simulink model "gm_HDL_pfc_gold_fi_vnl"  (R2024b)
settings: Solver=FixedStepDiscrete  StartTime=0.0  StopTime=.4  RelTol=1e-3
InitFcn:
  | fidelity_pfc_vals;
  | load('C:\Users\Angel\Desktop\hil\pfc3ph\matlab\sim\sschdl\pfc_desktop\stateSpaceParameters.mat');
undefined symbols (not defined in the file or in its folder): a, b, c, DiscIntNeverNeededParam, Down, Gs, s, stateSpaceParameters_1, t_ss, tsw, Up
libraries: simulink x32, hdlmdlgenlib x24, hdlsllib x8, eePwmGenerator x3, dspsrcs4 x3, hdlssclib x2, simulink_need_slupdate x1
(part 3 of 4)

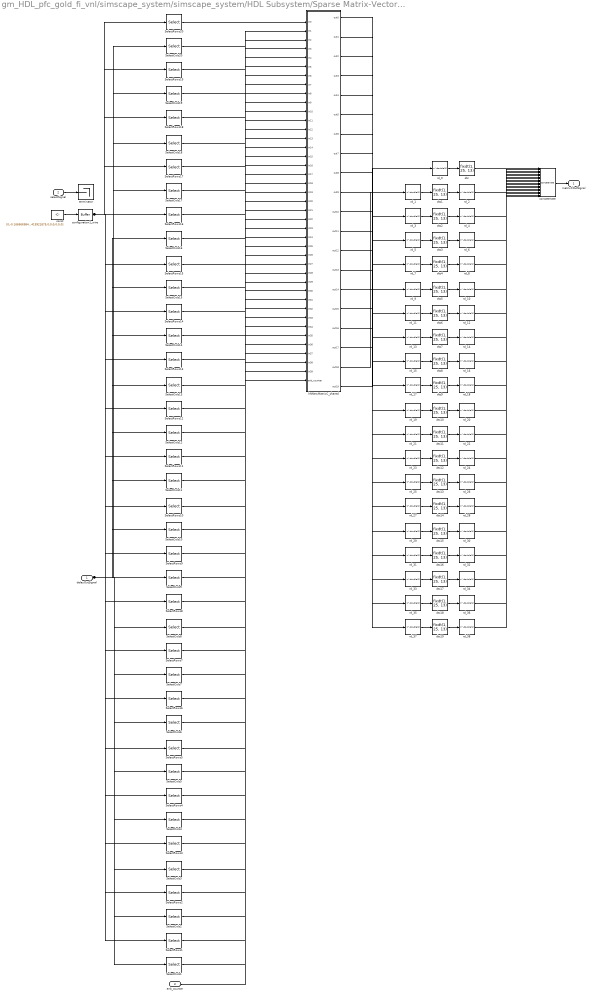
== system gm_HDL_pfc_gold_fi_vnl/simscape_system/simscape_system/HDL Subsystem/Sparse Matrix-Vector Product2 ==
  delayOutSignal : Inport  OutDataTypeStr=fixdt(1, 25, 13)  PortDimensions=[7]  SampleTime=7.65403750478377e-09
  selectSignal : Inport  Port=2  OutDataTypeStr=boolean  SampleTime=7.65403750478377e-09
  enb_counter : Inport  Port=3  OutDataTypeStr=fixdt(0, 7, 0)  SampleTime=7.65403750478377e-09
  SelectCols{1..20} (20 alike) : Selector  InputPortWidth=7  IndexOptions=Index vector (dialog)  Indices=double([1 2 3 4 5 6 7])  OutputSizes=double(1)
  SelectRows1 : Selector  InputPortWidth=140  IndexOptions=Index vector (dialog)  Indices=double([1 21 41 61 81 101 121])  OutputSizes=double(1)
  SelectRows10 : Selector  InputPortWidth=140  IndexOptions=Index vector (dialog)  Indices=double([10 30 50 70 90 110 130])  OutputSizes=double(1)
  SelectRows11 : Selector  InputPortWidth=140  IndexOptions=Index vector (dialog)  Indices=double([11 31 51 71 91 111 131])  OutputSizes=double(1)
  SelectRows12 : Selector  InputPortWidth=140  IndexOptions=Index vector (dialog)  Indices=double([12 32 52 72 92 112 132])  OutputSizes=double(1)
  SelectRows13 : Selector  InputPortWidth=140  IndexOptions=Index vector (dialog)  Indices=double([13 33 53 73 93 113 133])  OutputSizes=double(1)
  SelectRows14 : Selector  InputPortWidth=140  IndexOptions=Index vector (dialog)  Indices=double([14 34 54 74 94 114 134])  OutputSizes=double(1)
  SelectRows15 : Selector  InputPortWidth=140  IndexOptions=Index vector (dialog)  Indices=double([15 35 55 75 95 115 135])  OutputSizes=double(1)
  SelectRows16 : Selector  InputPortWidth=140  IndexOptions=Index vector (dialog)  Indices=double([16 36 56 76 96 116 136])  OutputSizes=double(1)
  SelectRows17 : Selector  InputPortWidth=140  IndexOptions=Index vector (dialog)  Indices=double([17 37 57 77 97 117 137])  OutputSizes=double(1)
  SelectRows18 : Selector  InputPortWidth=140  IndexOptions=Index vector (dialog)  Indices=double([18 38 58 78 98 118 138])  OutputSizes=double(1)
  SelectRows19 : Selector  InputPortWidth=140  IndexOptions=Index vector (dialog)  Indices=double([19 39 59 79 99 119 139])  OutputSizes=double(1)
  SelectRows2 : Selector  InputPortWidth=140  IndexOptions=Index vector (dialog)  Indices=double([2 22 42 62 82 102 122])  OutputSizes=double(1)
  SelectRows20 : Selector  InputPortWidth=140  IndexOptions=Index vector (dialog)  Indices=double([20 40 60 80 100 120 140])  OutputSizes=double(1)
  SelectRows3 : Selector  InputPortWidth=140  IndexOptions=Index vector (dialog)  Indices=double([3 23 43 63 83 103 123])  OutputSizes=double(1)
  SelectRows4 : Selector  InputPortWidth=140  IndexOptions=Index vector (dialog)  Indices=double([4 24 44 64 84 104 124])  OutputSizes=double(1)
  SelectRows5 : Selector  InputPortWidth=140  IndexOptions=Index vector (dialog)  Indices=double([5 25 45 65 85 105 125])  OutputSizes=double(1)
  SelectRows6 : Selector  InputPortWidth=140  IndexOptions=Index vector (dialog)  Indices=double([6 26 46 66 86 106 126])  OutputSizes=double(1)
  SelectRows7 : Selector  InputPortWidth=140  IndexOptions=Index vector (dialog)  Indices=double([7 27 47 67 87 107 127])  OutputSizes=double(1)
  SelectRows8 : Selector  InputPortWidth=140  IndexOptions=Index vector (dialog)  Indices=double([8 28 48 68 88 108 128])  OutputSizes=double(1)
  SelectRows9 : Selector  InputPortWidth=140  IndexOptions=Index vector (dialog)  Indices=double([9 29 49 69 89 109 129])  OutputSizes=double(1)
  concatenate : Concatenate  NumInputs=20
  configuration1_wire : hdlmdlgenlib/Buffer
  const : Constant  Value=[0;-0.16666698455810546875;-8.33333301544189453125;0.16666698455810546875;8.33333301544189453125;-0.08333301544189453125;-4.1666660308837890625;-0.08333301544189453125;-4.16666698455810546875;0.08333301544189453125;4.16666698455810546875;0.08333301544189453125;4.16666698455810546875;0;-0.16666698455810546875;-0.16666698455810546875;0.33333301544189453125;0;0;0;0;0.08333301544189453125;4.16666698455810546875;-0.08333301544189453125;-4.1666660308837890625;0.16666698455810546875;8.33333301544189453125;-0.08333301544189453125;-4.16666698455810546875;-0.16666698455810546875;-8.33333301544189453125;0.08333301544189453125;4.16666698455810546875;0;0.33333301544189453125;-0.16666698455810546875;-0.16666698455810546875;0;0;0;0;0.08333301544189453125;4.16666698455810546875;-0.08333301544189453125;-4.16666698455810546875;-0.08333301544189453125;-4.16666698455810546875;0.16666698455810546875;8.33333301544189453125;0.08333301544189453125;4.16666698455810546875;-0.16666698455810546875;-8.33333301544189453125;0;-0.16666698455810546875;0.33333301544189453125;-0.16666698455810546875;0;0;0;0;0.08333301544189453125;4.16666698455810546875;-0.08333301544189453125;-4.1666660308837890625;0.16666698455810546875;8.33333301544189453125;-0.08333301544189453125;-4.16666698455810546875;-0.16666698455810546875;-8.33333301544189453125;0.08333301544189453125;4.16666698455810546875;0;0.33333301544189453125;-0.16666698455810546875;-0.16666698455810546875;0;0;0;0;0.08333301544189453125;4.16666698455810546875;-0.08333301544189453125;-4.16666698455810546875;-0.08333301544189453125;-4.16666698455810546875;0.16666698455810546875;8.33333301544189453125;0.08333301544189453125;4.16666698455810546875;-0.16666698455810546875;-8.33333301544189453125;0;-0.16666698455810546875;0.33333301544189453125;-0.16666698455810546875;0;0;0;0;-0.16666698455810546875;-8.33333301544189453125;0.16666698455810546875;8.33333301544189453125;-0.08333301544189453125;-4.16666698455810546875;-0.08333301544189453125;-4.16666698455810546875;0.08333301544189453125;4.16666698455810546875;0.08333301544189453125;4.16666698455810546875;0;-0.16666698455810546875;-0.16666698455810546875;0.33333301544189453125;0;0;0;0;0.009998321533203125;0.4999103546142578125;0.009998321533203125;0.4999103546142578125;0.009998321533203125;0.4999103546142578125;0.009998321533203125;0.4999103546142578125;0.009998321533203125;0.4999103546142578125;0.009998321533203125;0.4999103546142578125;0.99981975555419921875;0;0;0;0;0;0]  OutDataTypeStr=fixdt(1, 25, 20)  SampleTime=7.65403750478377e-09
  dtc{,1..19} (20 alike) : DataTypeConversion  OutDataTypeStr=fixdt(1, 25, 13)  RndMeth=Nearest  SampleTime=7.65403750478377e-09  SaturateOnIntegerOverflow=off
  hNNewMatrixC_shared : Subsystem
  rd_{0..38} (39 alike) : Delay  DelayLength=double(1)  InitialCondition=0  SampleTime=7.65403750478377e-09
  terminator : Terminator
  matrixCOutSignal : Outport  OutDataTypeStr=fixdt(1, 25, 13)  PortDimensions=[20]  SampleTime=7.65403750478377e-09
  wires:
  hNNewMatrixC_shared/20(out19) -> rd_0/1
  selectSignal/1 -> terminator/1
  concatenate/1 -> matrixCOutSignal/1
  const/1 -> configuration1_wire/1
  SelectRows4/1 -> hNNewMatrixC_shared/33(in32)
  SelectRows5/1 -> hNNewMatrixC_shared/31(in30)
  SelectRows6/1 -> hNNewMatrixC_shared/29(in28)
  SelectRows8/1 -> hNNewMatrixC_shared/25(in24)
  SelectRows10/1 -> hNNewMatrixC_shared/21(in20)
  SelectRows11/1 -> hNNewMatrixC_shared/19(in18)
  SelectRows13/1 -> hNNewMatrixC_shared/15(in14)
  SelectRows14/1 -> hNNewMatrixC_shared/13(in12)
  SelectRows15/1 -> hNNewMatrixC_shared/11(in10)
  SelectRows17/1 -> hNNewMatrixC_shared/7(in6)
  SelectRows20/1 -> hNNewMatrixC_shared/1(in0)
  SelectCols2/1 -> hNNewMatrixC_shared/38(in37)
  SelectCols3/1 -> hNNewMatrixC_shared/36(in35)
  SelectCols4/1 -> hNNewMatrixC_shared/34(in33)
  SelectCols5/1 -> hNNewMatrixC_shared/32(in31)
  SelectCols6/1 -> hNNewMatrixC_shared/30(in29)
  SelectCols8/1 -> hNNewMatrixC_shared/26(in25)
  SelectRows19/1 -> hNNewMatrixC_shared/3(in2)
  SelectCols11/1 -> hNNewMatrixC_shared/20(in19)
  SelectCols13/1 -> hNNewMatrixC_shared/16(in15)
  SelectCols15/1 -> hNNewMatrixC_shared/12(in11)
  SelectCols16/1 -> hNNewMatrixC_shared/10(in9)
  SelectCols9/1 -> hNNewMatrixC_shared/24(in23)
  SelectCols18/1 -> hNNewMatrixC_shared/6(in5)
  SelectCols19/1 -> hNNewMatrixC_shared/4(in3)
  SelectCols20/1 -> hNNewMatrixC_shared/2(in1)
  hNNewMatrixC_shared/18(out17) -> rd_3/1
  SelectCols7/1 -> hNNewMatrixC_shared/28(in27)
  hNNewMatrixC_shared/17(out16) -> rd_5/1
  hNNewMatrixC_shared/16(out15) -> rd_7/1
  hNNewMatrixC_shared/15(out14) -> rd_9/1
  hNNewMatrixC_shared/13(out12) -> rd_13/1
  hNNewMatrixC_shared/12(out11) -> rd_15/1
  hNNewMatrixC_shared/11(out10) -> rd_17/1
  hNNewMatrixC_shared/10(out9) -> rd_19/1
  hNNewMatrixC_shared/9(out8) -> rd_21/1
  hNNewMatrixC_shared/8(out7) -> rd_23/1
  hNNewMatrixC_shared/7(out6) -> rd_25/1
  hNNewMatrixC_shared/6(out5) -> rd_27/1
  hNNewMatrixC_shared/5(out4) -> rd_29/1
  hNNewMatrixC_shared/3(out2) -> rd_33/1
  dtc/1 -> concatenate/1
  dtc1/1 -> rd_2/1
  hNNewMatrixC_shared/14(out13) -> rd_11/1
  SelectRows2/1 -> hNNewMatrixC_shared/37(in36)
  dtc2/1 -> rd_4/1
  dtc3/1 -> rd_6/1
  SelectCols14/1 -> hNNewMatrixC_shared/14(in13)
  dtc5/1 -> rd_10/1
  dtc6/1 -> rd_12/1
  dtc11/1 -> rd_22/1
  dtc7/1 -> rd_14/1
  SelectCols10/1 -> hNNewMatrixC_shared/22(in21)
  enb_counter/1 -> hNNewMatrixC_shared/41(enb_counter)
  rd_37/1 -> dtc19/1
  dtc10/1 -> rd_20/1
  SelectRows12/1 -> hNNewMatrixC_shared/17(in16)
  dtc15/1 -> rd_30/1
  hNNewMatrixC_shared/1(out0) -> rd_37/1
  rd_29/1 -> dtc15/1
  dtc19/1 -> rd_38/1
  dtc16/1 -> rd_32/1
  rd_19/1 -> dtc10/1
  dtc9/1 -> rd_18/1
  rd_15/1 -> dtc8/1
  rd_7/1 -> dtc4/1
  rd_13/1 -> dtc7/1
  rd_1/1 -> dtc1/1
  dtc12/1 -> rd_24/1
  rd_0/1 -> dtc/1
  dtc14/1 -> rd_28/1
  hNNewMatrixC_shared/19(out18) -> rd_1/1
  dtc13/1 -> rd_26/1
  rd_10/1 -> concatenate/6
  hNNewMatrixC_shared/2(out1) -> rd_35/1
  rd_17/1 -> dtc9/1
  dtc17/1 -> rd_34/1
  delayOutSignal/1 -> SelectCols9/1, SelectCols10/1, SelectCols11/1, SelectCols3/1, SelectCols15/1, SelectCols4/1, SelectCols7/1, SelectCols1/1, SelectCols2/1, SelectCols5/1, SelectCols6/1, SelectCols8/1, SelectCols12/1, SelectCols13/1, SelectCols14/1, SelectCols16/1, SelectCols17/1, SelectCols18/1, SelectCols19/1, SelectCols20/1
  dtc4/1 -> rd_8/1
  rd_12/1 -> concatenate/7
  SelectRows16/1 -> hNNewMatrixC_shared/9(in8)
  rd_23/1 -> dtc12/1
  rd_14/1 -> concatenate/8
  rd_9/1 -> dtc5/1
  rd_16/1 -> concatenate/9
  rd_3/1 -> dtc2/1
  rd_8/1 -> concatenate/5
  rd_20/1 -> concatenate/11
  SelectRows3/1 -> hNNewMatrixC_shared/35(in34)
  rd_35/1 -> dtc18/1
  SelectRows7/1 -> hNNewMatrixC_shared/27(in26)
  rd_31/1 -> dtc16/1
  rd_26/1 -> concatenate/14
  rd_4/1 -> concatenate/3
  SelectRows9/1 -> hNNewMatrixC_shared/23(in22)
  rd_5/1 -> dtc3/1
  rd_33/1 -> dtc17/1
  SelectRows1/1 -> hNNewMatrixC_shared/39(in38)
  rd_11/1 -> dtc6/1
  rd_25/1 -> dtc13/1
  rd_30/1 -> concatenate/16
  SelectCols17/1 -> hNNewMatrixC_shared/8(in7)
  rd_32/1 -> concatenate/17
  rd_24/1 -> concatenate/13
  rd_36/1 -> concatenate/19
  rd_22/1 -> concatenate/12
  SelectCols1/1 -> hNNewMatrixC_shared/40(in39)
  rd_2/1 -> concatenate/2
  rd_21/1 -> dtc11/1
  rd_27/1 -> dtc14/1
  rd_18/1 -> concatenate/10
  SelectRows18/1 -> hNNewMatrixC_shared/5(in4)
  rd_28/1 -> concatenate/15
  dtc18/1 -> rd_36/1
  SelectCols12/1 -> hNNewMatrixC_shared/18(in17)
  configuration1_wire/1 -> SelectRows12/1, SelectRows17/1, SelectRows13/1, SelectRows2/1, SelectRows15/1, SelectRows20/1, SelectRows10/1, SelectRows5/1, SelectRows1/1, SelectRows3/1, SelectRows4/1, SelectRows6/1, SelectRows7/1, SelectRows8/1, SelectRows9/1, SelectRows11/1, SelectRows14/1, SelectRows16/1, SelectRows18/1, SelectRows19/1
  rd_6/1 -> concatenate/4
  dtc8/1 -> rd_16/1
  rd_34/1 -> concatenate/18
  hNNewMatrixC_shared/4(out3) -> rd_31/1
  rd_38/1 -> concatenate/20

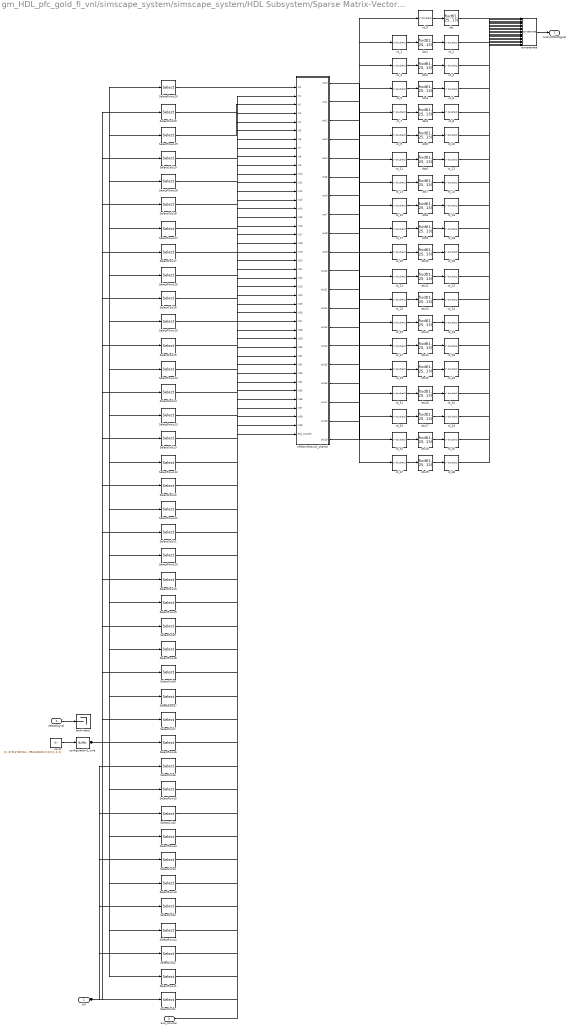
== system gm_HDL_pfc_gold_fi_vnl/simscape_system/simscape_system/HDL Subsystem/Sparse Matrix-Vector Product3 ==
  in0 : Inport  OutDataTypeStr=fixdt(1, 25, 13)  PortDimensions=[10]  SampleTime=7.65403750478377e-09
  selectSignal : Inport  Port=2  OutDataTypeStr=boolean  SampleTime=7.65403750478377e-09
  enb_counter : Inport  Port=3  OutDataTypeStr=fixdt(0, 7, 0)  SampleTime=7.65403750478377e-09
  SelectCols{1..17} (17 alike) : Selector  InputPortWidth=10  IndexOptions=Index vector (dialog)  Indices=double([1 2 3 4 5 6 7])  OutputSizes=double(1)
  SelectCols18 : Selector  InputPortWidth=10  IndexOptions=Index vector (dialog)  Indices=double([1 2 3 4 5 6 9])  OutputSizes=double(1)
  SelectCols19 : Selector  InputPortWidth=10  IndexOptions=Index vector (dialog)  Indices=double([1 2 3 4 5 6 10])  OutputSizes=double(1)
  SelectCols20 : Selector  InputPortWidth=10  IndexOptions=Index vector (dialog)  Indices=double([1 2 3 4 5 6 8])  OutputSizes=double(1)
  SelectRows1 : Selector  InputPortWidth=140  IndexOptions=Index vector (dialog)  Indices=double([1 21 41 61 81 101 121])  OutputSizes=double(1)
  SelectRows10 : Selector  InputPortWidth=140  IndexOptions=Index vector (dialog)  Indices=double([10 30 50 70 90 110 130])  OutputSizes=double(1)
  SelectRows11 : Selector  InputPortWidth=140  IndexOptions=Index vector (dialog)  Indices=double([11 31 51 71 91 111 131])  OutputSizes=double(1)
  SelectRows12 : Selector  InputPortWidth=140  IndexOptions=Index vector (dialog)  Indices=double([12 32 52 72 92 112 132])  OutputSizes=double(1)
  SelectRows13 : Selector  InputPortWidth=140  IndexOptions=Index vector (dialog)  Indices=double([13 33 53 73 93 113 133])  OutputSizes=double(1)
  SelectRows14 : Selector  InputPortWidth=140  IndexOptions=Index vector (dialog)  Indices=double([14 34 54 74 94 114 134])  OutputSizes=double(1)
  SelectRows15 : Selector  InputPortWidth=140  IndexOptions=Index vector (dialog)  Indices=double([15 35 55 75 95 115 135])  OutputSizes=double(1)
  SelectRows16 : Selector  InputPortWidth=140  IndexOptions=Index vector (dialog)  Indices=double([16 36 56 76 96 116 136])  OutputSizes=double(1)
  SelectRows17 : Selector  InputPortWidth=140  IndexOptions=Index vector (dialog)  Indices=double([17 37 57 77 97 117 137])  OutputSizes=double(1)
  SelectRows18 : Selector  InputPortWidth=140  IndexOptions=Index vector (dialog)  Indices=double([18 38 58 78 98 118 139])  OutputSizes=double(1)
  SelectRows19 : Selector  InputPortWidth=140  IndexOptions=Index vector (dialog)  Indices=double([19 39 59 79 99 119 140])  OutputSizes=double(1)
  SelectRows2 : Selector  InputPortWidth=140  IndexOptions=Index vector (dialog)  Indices=double([2 22 42 62 82 102 122])  OutputSizes=double(1)
  SelectRows20 : Selector  InputPortWidth=140  IndexOptions=Index vector (dialog)  Indices=double([20 40 60 80 100 120 138])  OutputSizes=double(1)
  SelectRows3 : Selector  InputPortWidth=140  IndexOptions=Index vector (dialog)  Indices=double([3 23 43 63 83 103 123])  OutputSizes=double(1)
  SelectRows4 : Selector  InputPortWidth=140  IndexOptions=Index vector (dialog)  Indices=double([4 24 44 64 84 104 124])  OutputSizes=double(1)
  SelectRows5 : Selector  InputPortWidth=140  IndexOptions=Index vector (dialog)  Indices=double([5 25 45 65 85 105 125])  OutputSizes=double(1)
  SelectRows6 : Selector  InputPortWidth=140  IndexOptions=Index vector (dialog)  Indices=double([6 26 46 66 86 106 126])  OutputSizes=double(1)
  SelectRows7 : Selector  InputPortWidth=140  IndexOptions=Index vector (dialog)  Indices=double([7 27 47 67 87 107 127])  OutputSizes=double(1)
  SelectRows8 : Selector  InputPortWidth=140  IndexOptions=Index vector (dialog)  Indices=double([8 28 48 68 88 108 128])  OutputSizes=double(1)
  SelectRows9 : Selector  InputPortWidth=140  IndexOptions=Index vector (dialog)  Indices=double([9 29 49 69 89 109 129])  OutputSizes=double(1)
  concatenate : Concatenate  NumInputs=20
  configuration1_wire : hdlmdlgenlib/Buffer
  const : Constant  Value=[1;-5.91278076171875e-05;-0.0030002593994140625;-5.91278076171875e-05;-0.0030002593994140625;-5.91278076171875e-05;-0.0030002593994140625;-5.91278076171875e-05;-0.0030002593994140625;-5.91278076171875e-05;-0.0030002593994140625;-5.91278076171875e-05;-0.0030002593994140625;-0.0059986114501953125;0;0;0;0;0;0;0;-0.499969482421875;25.001499176025390625;-0.499969482421875;-24.998500823974609375;3.0517578125e-05;0.001499176025390625;3.0517578125e-05;0.001499176025390625;3.0517578125e-05;0.001499176025390625;3.0517578125e-05;0.001499176025390625;0.0030002593994140625;0;0;0;0;0;0;0;-0.499969482421875;-24.998500823974609375;-0.499969482421875;25.001499176025390625;3.0517578125e-05;0.001499176025390625;3.0517578125e-05;0.001499176025390625;3.0517578125e-05;0.001499176025390625;3.0517578125e-05;0.001499176025390625;0.0030002593994140625;0;0;0;0;0;0;0;3.0517578125e-05;0.001499176025390625;3.0517578125e-05;0.001499176025390625;-0.499969482421875;25.001499176025390625;3.0517578125e-05;0.001499176025390625;-0.499969482421875;-24.998500823974609375;3.0517578125e-05;0.001499176025390625;0.0030002593994140625;0;0;0;0;0;0;0;3.0517578125e-05;0.001499176025390625;3.0517578125e-05;0.001499176025390625;3.0517578125e-05;0.001499176025390625;-0.499969482421875;25.001499176025390625;3.0517578125e-05;0.001499176025390625;-0.499969482421875;-24.998500823974609375;0.0030002593994140625;0;0;0;0;0;0;0;3.0517578125e-05;0.001499176025390625;3.0517578125e-05;0.001499176025390625;-0.499969482421875;-24.998500823974609375;3.0517578125e-05;0.001499176025390625;-0.499969482421875;25.001499176025390625;3.0517578125e-05;0.001499176025390625;0.0030002593994140625;0;0;0;0;0;0;0;3.0517578125e-05;0.001499176025390625;3.0517578125e-05;0.001499176025390625;3.0517578125e-05;0.001499176025390625;-0.499969482421875;-24.998500823974609375;3.0517578125e-05;0.001499176025390625;-0.499969482421875;25.001499176025390625;0.0030002593994140625;0;0;0;1;1;1]  OutDataTypeStr=fixdt(1, 25, 19)  SampleTime=7.65403750478377e-09
  dtc{,1..19} (20 alike) : DataTypeConversion  OutDataTypeStr=fixdt(1, 25, 13)  RndMeth=Nearest  SampleTime=7.65403750478377e-09  SaturateOnIntegerOverflow=off
  hNNewMatrixD_shared : Subsystem
  rd_{0..38} (39 alike) : Delay  DelayLength=double(1)  InitialCondition=0  SampleTime=7.65403750478377e-09
  terminator : Terminator
  matrixDOutSignal : Outport  OutDataTypeStr=fixdt(1, 25, 13)  PortDimensions=[20]  SampleTime=7.65403750478377e-09
  wires:
  hNNewMatrixD_shared/20(out19) -> rd_0/1
  selectSignal/1 -> terminator/1
  concatenate/1 -> matrixDOutSignal/1
  const/1 -> configuration1_wire/1
  SelectRows3/1 -> hNNewMatrixD_shared/35(in34)
  SelectRows4/1 -> hNNewMatrixD_shared/33(in32)
  SelectRows5/1 -> hNNewMatrixD_shared/31(in30)
  SelectRows7/1 -> hNNewMatrixD_shared/27(in26)
  SelectRows9/1 -> hNNewMatrixD_shared/23(in22)
  SelectRows10/1 -> hNNewMatrixD_shared/21(in20)
  SelectRows11/1 -> hNNewMatrixD_shared/19(in18)
  SelectRows15/1 -> hNNewMatrixD_shared/11(in10)
  SelectRows17/1 -> hNNewMatrixD_shared/7(in6)
  SelectRows18/1 -> hNNewMatrixD_shared/5(in4)
  SelectRows19/1 -> hNNewMatrixD_shared/3(in2)
  SelectRows20/1 -> hNNewMatrixD_shared/1(in0)
  SelectCols2/1 -> hNNewMatrixD_shared/38(in37)
  SelectCols3/1 -> hNNewMatrixD_shared/36(in35)
  SelectCols4/1 -> hNNewMatrixD_shared/34(in33)
  SelectCols5/1 -> hNNewMatrixD_shared/32(in31)
  SelectCols6/1 -> hNNewMatrixD_shared/30(in29)
  SelectCols7/1 -> hNNewMatrixD_shared/28(in27)
  SelectCols8/1 -> hNNewMatrixD_shared/26(in25)
  SelectCols11/1 -> hNNewMatrixD_shared/20(in19)
  SelectCols13/1 -> hNNewMatrixD_shared/16(in15)
  SelectCols14/1 -> hNNewMatrixD_shared/14(in13)
  SelectCols15/1 -> hNNewMatrixD_shared/12(in11)
  SelectCols16/1 -> hNNewMatrixD_shared/10(in9)
  SelectCols12/1 -> hNNewMatrixD_shared/18(in17)
  SelectCols20/1 -> hNNewMatrixD_shared/2(in1)
  hNNewMatrixD_shared/17(out16) -> rd_5/1
  SelectRows16/1 -> hNNewMatrixD_shared/9(in8)
  hNNewMatrixD_shared/16(out15) -> rd_7/1
  hNNewMatrixD_shared/15(out14) -> rd_9/1
  hNNewMatrixD_shared/14(out13) -> rd_11/1
  SelectRows6/1 -> hNNewMatrixD_shared/29(in28)
  configuration1_wire/1 -> SelectRows2/1, SelectRows11/1, SelectRows18/1, SelectRows9/1, SelectRows8/1, SelectRows1/1, SelectRows3/1, SelectRows4/1, SelectRows5/1, SelectRows6/1, SelectRows7/1, SelectRows10/1, SelectRows12/1, SelectRows13/1, SelectRows14/1, SelectRows15/1, SelectRows16/1, SelectRows17/1, SelectRows19/1, SelectRows20/1
  SelectCols1/1 -> hNNewMatrixD_shared/40(in39)
  hNNewMatrixD_shared/11(out10) -> rd_17/1
  hNNewMatrixD_shared/9(out8) -> rd_21/1
  hNNewMatrixD_shared/8(out7) -> rd_23/1
  hNNewMatrixD_shared/7(out6) -> rd_25/1
  hNNewMatrixD_shared/6(out5) -> rd_27/1
  SelectCols19/1 -> hNNewMatrixD_shared/4(in3)
  hNNewMatrixD_shared/5(out4) -> rd_29/1
  SelectCols18/1 -> hNNewMatrixD_shared/6(in5)
  hNNewMatrixD_shared/4(out3) -> rd_31/1
  hNNewMatrixD_shared/2(out1) -> rd_35/1
  dtc1/1 -> rd_2/1
  dtc4/1 -> rd_8/1
  dtc8/1 -> rd_16/1
  hNNewMatrixD_shared/1(out0) -> rd_37/1
  dtc13/1 -> rd_26/1
  dtc16/1 -> rd_32/1
  dtc19/1 -> rd_38/1
  SelectRows13/1 -> hNNewMatrixD_shared/15(in14)
  dtc14/1 -> rd_28/1
  rd_15/1 -> dtc8/1
  rd_37/1 -> dtc19/1
  rd_1/1 -> dtc1/1
  rd_13/1 -> dtc7/1
  rd_35/1 -> dtc18/1
  hNNewMatrixD_shared/12(out11) -> rd_15/1
  rd_25/1 -> dtc13/1
  rd_29/1 -> dtc15/1
  hNNewMatrixD_shared/3(out2) -> rd_33/1
  SelectRows8/1 -> hNNewMatrixD_shared/25(in24)
  dtc18/1 -> rd_36/1
  rd_4/1 -> concatenate/3
  rd_3/1 -> dtc2/1
  rd_19/1 -> dtc10/1
  SelectCols9/1 -> hNNewMatrixD_shared/24(in23)
  rd_6/1 -> concatenate/4
  rd_31/1 -> dtc16/1
  rd_0/1 -> dtc/1
  rd_23/1 -> dtc12/1
  dtc12/1 -> rd_24/1
  SelectRows14/1 -> hNNewMatrixD_shared/13(in12)
  rd_8/1 -> concatenate/5
  rd_10/1 -> concatenate/6
  rd_21/1 -> dtc11/1
  dtc5/1 -> rd_10/1
  SelectRows12/1 -> hNNewMatrixD_shared/17(in16)
  rd_12/1 -> concatenate/7
  rd_33/1 -> dtc17/1
  SelectCols10/1 -> hNNewMatrixD_shared/22(in21)
  dtc2/1 -> rd_4/1
  in0/1 -> SelectCols20/1, SelectCols3/1, SelectCols15/1, SelectCols19/1, SelectCols1/1, SelectCols2/1, SelectCols4/1, SelectCols5/1, SelectCols6/1, SelectCols7/1, SelectCols8/1, SelectCols11/1, SelectCols9/1, SelectCols10/1, SelectCols12/1, SelectCols13/1, SelectCols14/1, SelectCols16/1, SelectCols17/1, SelectCols18/1
  dtc15/1 -> rd_30/1
  rd_18/1 -> concatenate/10
  rd_2/1 -> concatenate/2
  hNNewMatrixD_shared/19(out18) -> rd_1/1
  dtc7/1 -> rd_14/1
  enb_counter/1 -> hNNewMatrixD_shared/41(enb_counter)
  rd_20/1 -> concatenate/11
  rd_28/1 -> concatenate/15
  rd_9/1 -> dtc5/1
  rd_32/1 -> concatenate/17
  hNNewMatrixD_shared/18(out17) -> rd_3/1
  dtc10/1 -> rd_20/1
  rd_11/1 -> dtc6/1
  rd_5/1 -> dtc3/1
  rd_27/1 -> dtc14/1
  dtc17/1 -> rd_34/1
  rd_34/1 -> concatenate/18
  dtc11/1 -> rd_22/1
  dtc/1 -> concatenate/1
  rd_26/1 -> concatenate/14
  dtc3/1 -> rd_6/1
  rd_17/1 -> dtc9/1
  dtc9/1 -> rd_18/1
  rd_24/1 -> concatenate/13
  rd_14/1 -> concatenate/8
  hNNewMatrixD_shared/10(out9) -> rd_19/1
  rd_36/1 -> concatenate/19
  hNNewMatrixD_shared/13(out12) -> rd_13/1
  rd_16/1 -> concatenate/9
  dtc6/1 -> rd_12/1
  SelectRows1/1 -> hNNewMatrixD_shared/39(in38)
  rd_30/1 -> concatenate/16
  rd_7/1 -> dtc4/1
  rd_22/1 -> concatenate/12
  SelectCols17/1 -> hNNewMatrixD_shared/8(in7)
  rd_38/1 -> concatenate/20
  SelectRows2/1 -> hNNewMatrixD_shared/37(in36)

== system gm_HDL_pfc_gold_fi_vnl/simscape_system_vnl/HDL Subsystem/HDL Algorithm/Output ==
  In1 : Inport
  State : Inport  Port=2
  Sel : Inport  Port=3  LockScale=on
  Bias : Terminator
  Mux : Mux  Inputs=2
  Output Update : hdlssclib/NFPSparseConstMultiply  MatrixSource=Dialog  constMatrix=single([stateSpaceParameters_1.Cd stateSpaceParameters_1.Dd])  MatrixType=single  MatrixSize=[1 1]  ColumnIndices=[1]  RowIndices=[1]  PropDataType=single  defWL=48
  Out1 : Outport  VectorParamsAs1DForOutWhenUnconnected=off
  wires:
  Output Update/1 -> Out1/1
  Sel/1 -> Output Update/2, Bias/1
  In1/1 -> Mux/2
  Mux/1 -> Output Update/1
  State/1 -> Mux/1

== system gm_HDL_pfc_gold_fi_vnl/simscape_system_vnl/HDL Subsystem/HDL Algorithm/State Update ==
  In1 : Inport
  State : Inport  Port=2
  Sel : Inport  Port=3  LockScale=on
  Bias : Terminator
  Mux : Mux  Inputs=2
  State Update : hdlssclib/NFPSparseConstMultiply  MatrixSource=Dialog  constMatrix=single([stateSpaceParameters_1.Ad stateSpaceParameters_1.Bd])  MatrixType=single  MatrixSize=[1 1]  ColumnIndices=[1]  RowIndices=[1]  PropDataType=single  defWL=43
  State Out : Outport  VectorParamsAs1DForOutWhenUnconnected=off
  wires:
  State Update/1 -> State Out/1
  Sel/1 -> State Update/2, Bias/1
  Mux/1 -> State Update/1
  In1/1 -> Mux/2
  State/1 -> Mux/1

== system gm_HDL_pfc_gold_fi_vnl/simscape_system/simscape_system/FET_CTRL/crp_temp_shared/Gain3_out1_bypass ==
  in0 : Inport  OutDataTypeStr=fixdt(1, 36, 0)  PortDimensions=[6]  SampleTime=7.65403750478377e-09
  in1 : Inport  Port=2  OutDataTypeStr=boolean  SampleTime=7.65403750478377e-09
  Gain3_out1_enb : Switch  Criteria=u2 ~= 0  Threshold=double(0)  OutDataTypeStr=fixdt(1, 36, 0)  SampleTime=7.65403750478377e-09  SaturateOnIntegerOverflow=off  InputSameDT=off
  Gain3_out1_state : Delay  DelayLength=double(1)  InitialCondition=0  SampleTime=7.65403750478377e-09
  out0 : Outport  OutDataTypeStr=fixdt(1, 36, 0)  PortDimensions=[6]  SampleTime=7.65403750478377e-09
  wires:
  Gain3_out1_state/1 -> Gain3_out1_enb/3
  in1/1 -> Gain3_out1_enb/2
  Gain3_out1_enb/1 -> out0/1, Gain3_out1_state/1
  in0/1 -> Gain3_out1_enb/1

== system gm_HDL_pfc_gold_fi_vnl/simscape_system/simscape_system/FET_CTRL/crp_temp_shared/Serializer_Subnetwork ==
  in0 : Inport  OutDataTypeStr=fixdt(1, 18, 0)  PortDimensions=[12]  SampleTime=7.65403750478377e-09
  in1 : Inport  Port=2  OutDataTypeStr=fixdt(0, 1, 0)  SampleTime=7.65403750478377e-09
  ratechange_splitcomp : Demux  Outputs=2
  splitcomp_multiport : MultiPortSwitch  DataPortOrder=Zero-based contiguous  Inputs=2  DiagnosticForDefault=None  zeroidx=on  OutDataTypeStr=fixdt(1, 18, 0)  SampleTime=7.65403750478377e-09  SaturateOnIntegerOverflow=off  InputSameDT=off
  out0 : Outport  OutDataTypeStr=fixdt(1, 18, 0)  PortDimensions=[6]  SampleTime=7.65403750478377e-09
  wires:
  splitcomp_multiport/1 -> out0/1
  ratechange_splitcomp/1 -> splitcomp_multiport/2
  in1/1 -> splitcomp_multiport/1
  ratechange_splitcomp/2 -> splitcomp_multiport/3
  in0/1 -> ratechange_splitcomp/1

== system gm_HDL_pfc_gold_fi_vnl/simscape_system/simscape_system/FET_CTRL/crp_temp_shared/Serializer_Subnetwork1 ==
  in0 : Inport  OutDataTypeStr=fixdt(1, 18, 0)  PortDimensions=[2]  SampleTime=7.65403750478377e-09
  in1 : Inport  Port=2  OutDataTypeStr=fixdt(0, 1, 0)  SampleTime=7.65403750478377e-09
  ratechange_splitcomp : Demux  Outputs=2
  splitcomp_multiport : MultiPortSwitch  DataPortOrder=Zero-based contiguous  Inputs=2  DiagnosticForDefault=None  zeroidx=on  OutDataTypeStr=fixdt(1, 18, 0)  SampleTime=7.65403750478377e-09  SaturateOnIntegerOverflow=off  InputSameDT=off
  out0 : Outport  OutDataTypeStr=fixdt(1, 18, 0)  SampleTime=7.65403750478377e-09
  wires:
  splitcomp_multiport/1 -> out0/1
  ratechange_splitcomp/2 -> splitcomp_multiport/3
  ratechange_splitcomp/1 -> splitcomp_multiport/2
  in0/1 -> ratechange_splitcomp/1
  in1/1 -> splitcomp_multiport/1

== system gm_HDL_pfc_gold_fi_vnl/simscape_system/simscape_system/FET_CTRL/crp_temp_shared/counter ==
  globalSchedule : EnablePort  OutDataTypeStr=boolean
  ctr_0_1 : hdlsllib/Sources/HDL Counter  CountType=Count limited  CountInit=double(0)  CountStep=double(1)  CountMax=double(1)  CountFromType=Initial value  CountFrom=double(0)  CountResetPort=off  CountLoadPort=off  CountEnbPort=off  CountDirPort=off  CountHitOutputPort=off  CountDataType=Unsigned  CountWordLen=1  CountFracLen=0  CountSampTime=7.65403750478377e-09
  out0 : Outport  OutDataTypeStr=fixdt(0, 1, 0)  SampleTime=7.65403750478377e-09  InitialOutput=0
  wires:
  ctr_0_1/1 -> out0/1

== system gm_HDL_pfc_gold_fi_vnl/simscape_system/simscape_system/HDL Subsystem/Sparse Matrix-Vector Product/hNNewMatrixB_shared ==
  in0 : Inport  OutDataTypeStr=fixdt(1, 25, 31)  PortDimensions=[9]  SampleTime=7.65403750478377e-09
  in1 : Inport  Port=2  OutDataTypeStr=fixdt(1, 25, 13)  PortDimensions=[9]  SampleTime=7.65403750478377e-09
  in2 : Inport  Port=3  OutDataTypeStr=fixdt(1, 25, 31)  PortDimensions=[9]  SampleTime=7.65403750478377e-09
  in3 : Inport  Port=4  OutDataTypeStr=fixdt(1, 25, 13)  PortDimensions=[9]  SampleTime=7.65403750478377e-09
  in4 : Inport  Port=5  OutDataTypeStr=fixdt(1, 25, 31)  PortDimensions=[9]  SampleTime=7.65403750478377e-09
  in5 : Inport  Port=6  OutDataTypeStr=fixdt(1, 25, 13)  PortDimensions=[9]  SampleTime=7.65403750478377e-09
  in6 : Inport  Port=7  OutDataTypeStr=fixdt(1, 25, 31)  PortDimensions=[9]  SampleTime=7.65403750478377e-09
  in7 : Inport  Port=8  OutDataTypeStr=fixdt(1, 25, 13)  PortDimensions=[9]  SampleTime=7.65403750478377e-09
  in8 : Inport  Port=9  OutDataTypeStr=fixdt(1, 25, 31)  PortDimensions=[9]  SampleTime=7.65403750478377e-09
  in9 : Inport  Port=10  OutDataTypeStr=fixdt(1, 25, 13)  PortDimensions=[9]  SampleTime=7.65403750478377e-09
  in10 : Inport  Port=11  OutDataTypeStr=fixdt(1, 25, 31)  PortDimensions=[9]  SampleTime=7.65403750478377e-09
  in11 : Inport  Port=12  OutDataTypeStr=fixdt(1, 25, 13)  PortDimensions=[9]  SampleTime=7.65403750478377e-09
  in12 : Inport  Port=13  OutDataTypeStr=fixdt(1, 25, 31)  PortDimensions=[9]  SampleTime=7.65403750478377e-09
  in13 : Inport  Port=14  OutDataTypeStr=fixdt(1, 25, 13)  PortDimensions=[9]  SampleTime=7.65403750478377e-09
  enb_counter : Inport  Port=15  OutDataTypeStr=fixdt(0, 7, 0)  SampleTime=7.65403750478377e-09
  Serializer_Subnetwork : Subsystem
  Serializer_Subnetwork1 : Subsystem
  counter : Subsystem
  demux : Demux  Outputs=6
  dot_product1_bypass : Subsystem
  dot_product_9 : Subsystem
  enb_counter_eq_8 : simulink/Logic and Bit Operations/Compare To Constant  relop===  const=double(8)  OutDataTypeStr=boolean
  enb_counter_ge_2 : simulink/Logic and Bit Operations/Compare To Constant  relop=>=  const=double(2)  OutDataTypeStr=boolean
  enb_counter_ge_2_and_enb_counter_le_7 : Logic  AllPortsSameDT=off  OutDataTypeStr=boolean  SampleTime=7.65403750478377e-09
  enb_counter_le_6 : simulink/Logic and Bit Operations/Compare To Constant  relop=<=  const=double(6)  OutDataTypeStr=boolean
  enb_counter_le_7 : simulink/Logic and Bit Operations/Compare To Constant  relop=<=  const=double(7)  OutDataTypeStr=boolean
  mux : Mux  Inputs=7
  mux1 : Mux  Inputs=7
  rd_{0..2,4} (4 alike) : Delay  DelayLength=double(1)  InitialCondition=0  SampleTime=7.65403750478377e-09
  rd_3 : Delay  DelayLength=double(4)  InitialCondition=0  SampleTime=7.65403750478377e-09
  rd_5 : Delay  DelayLength=double(6)  InitialCondition=0  SampleTime=7.65403750478377e-09
  tappedDelay : Subsystem
  out0 : Outport  OutDataTypeStr=fixdt(1, 50, 44)  SampleTime=7.65403750478377e-09
  out1 : Outport  Port=2  OutDataTypeStr=fixdt(1, 50, 44)  SampleTime=7.65403750478377e-09
  out2 : Outport  Port=3  OutDataTypeStr=fixdt(1, 50, 44)  SampleTime=7.65403750478377e-09
  out3 : Outport  Port=4  OutDataTypeStr=fixdt(1, 50, 44)  SampleTime=7.65403750478377e-09
  out4 : Outport  Port=5  OutDataTypeStr=fixdt(1, 50, 44)  SampleTime=7.65403750478377e-09
  out5 : Outport  Port=6  OutDataTypeStr=fixdt(1, 50, 44)  SampleTime=7.65403750478377e-09
  out6 : Outport  Port=7  OutDataTypeStr=fixdt(1, 50, 44)  SampleTime=7.65403750478377e-09
  wires:
  demux/3 -> out2/1
  demux/5 -> out4/1
  demux/2 -> out1/1
  rd_4/1 -> dot_product1_bypass/1(in0)
  dot_product_9/1(out1) -> tappedDelay/1(in0), rd_4/1
  rd_3/1 -> tappedDelay/Enable
  Serializer_Subnetwork1/1(out0) -> dot_product_9/2(in2)
  mux1/1 -> Serializer_Subnetwork1/1(in0)
  mux/1 -> Serializer_Subnetwork/1(in0)
  enb_counter_ge_2_and_enb_counter_le_7/1 -> rd_3/1
  in13/1 -> mux1/7
  in11/1 -> mux1/6
  in9/1 -> mux1/5
  rd_5/1 -> dot_product1_bypass/2(in1)
  in5/1 -> mux1/3
  in3/1 -> mux1/2
  in1/1 -> mux1/1
  rd_0/1 -> counter/Enable
  in12/1 -> mux/7
  demux/6 -> out5/1
  in10/1 -> mux/6
  in8/1 -> mux/5
  tappedDelay/1(out0) -> demux/1
  dot_product1_bypass/1(out0) -> out6/1
  in6/1 -> mux/4
  Serializer_Subnetwork/1(out0) -> dot_product_9/1(in1)
  in4/1 -> mux/3
  in2/1 -> mux/2
  rd_2/1 -> enb_counter_ge_2_and_enb_counter_le_7/2
  enb_counter_le_7/1 -> rd_2/1
  in7/1 -> mux1/4
  demux/4 -> out3/1
  in0/1 -> mux/1
  enb_counter_le_6/1 -> rd_0/1
  enb_counter_ge_2/1 -> rd_1/1
  rd_1/1 -> enb_counter_ge_2_and_enb_counter_le_7/1
  counter/1(out0) -> Serializer_Subnetwork/2(in1), Serializer_Subnetwork1/2(in1)
  enb_counter/1 -> enb_counter_le_6/1, enb_counter_le_7/1, enb_counter_ge_2/1, enb_counter_eq_8/1
  demux/1 -> out0/1
  enb_counter_eq_8/1 -> rd_5/1

== system gm_HDL_pfc_gold_fi_vnl/simscape_system/simscape_system/HDL Subsystem/Sparse Matrix-Vector Product1/hNNewMatrixA_shared ==
  in0 : Inport  OutDataTypeStr=fixdt(1, 25, 24)  PortDimensions=[6]  SampleTime=7.65403750478377e-09
  in1 : Inport  Port=2  OutDataTypeStr=fixdt(1, 25, 13)  PortDimensions=[6]  SampleTime=7.65403750478377e-09
  in2 : Inport  Port=3  OutDataTypeStr=fixdt(1, 25, 24)  PortDimensions=[6]  SampleTime=7.65403750478377e-09
  in3 : Inport  Port=4  OutDataTypeStr=fixdt(1, 25, 13)  PortDimensions=[6]  SampleTime=7.65403750478377e-09
  in4 : Inport  Port=5  OutDataTypeStr=fixdt(1, 25, 24)  PortDimensions=[6]  SampleTime=7.65403750478377e-09
  in5 : Inport  Port=6  OutDataTypeStr=fixdt(1, 25, 13)  PortDimensions=[6]  SampleTime=7.65403750478377e-09
  in6 : Inport  Port=7  OutDataTypeStr=fixdt(1, 25, 24)  PortDimensions=[6]  SampleTime=7.65403750478377e-09
  in7 : Inport  Port=8  OutDataTypeStr=fixdt(1, 25, 13)  PortDimensions=[6]  SampleTime=7.65403750478377e-09
  in8 : Inport  Port=9  OutDataTypeStr=fixdt(1, 25, 24)  PortDimensions=[6]  SampleTime=7.65403750478377e-09
  in9 : Inport  Port=10  OutDataTypeStr=fixdt(1, 25, 13)  PortDimensions=[6]  SampleTime=7.65403750478377e-09
  in10 : Inport  Port=11  OutDataTypeStr=fixdt(1, 25, 24)  PortDimensions=[6]  SampleTime=7.65403750478377e-09
  in11 : Inport  Port=12  OutDataTypeStr=fixdt(1, 25, 13)  PortDimensions=[6]  SampleTime=7.65403750478377e-09
  in12 : Inport  Port=13  OutDataTypeStr=fixdt(1, 25, 24)  PortDimensions=[6]  SampleTime=7.65403750478377e-09
  in13 : Inport  Port=14  OutDataTypeStr=fixdt(1, 25, 13)  PortDimensions=[6]  SampleTime=7.65403750478377e-09
  enb_counter : Inport  Port=15  OutDataTypeStr=fixdt(0, 7, 0)  SampleTime=7.65403750478377e-09
  Serializer_Subnetwork : Subsystem
  Serializer_Subnetwork1 : Subsystem
  counter : Subsystem
  demux : Demux  Outputs=6
  dot_product1_bypass : Subsystem
  dot_product_6 : Subsystem
  enb_counter_eq_8 : simulink/Logic and Bit Operations/Compare To Constant  relop===  const=double(8)  OutDataTypeStr=boolean
  enb_counter_ge_2 : simulink/Logic and Bit Operations/Compare To Constant  relop=>=  const=double(2)  OutDataTypeStr=boolean
  enb_counter_ge_2_and_enb_counter_le_7 : Logic  AllPortsSameDT=off  OutDataTypeStr=boolean  SampleTime=7.65403750478377e-09
  enb_counter_le_6 : simulink/Logic and Bit Operations/Compare To Constant  relop=<=  const=double(6)  OutDataTypeStr=boolean
  enb_counter_le_7 : simulink/Logic and Bit Operations/Compare To Constant  relop=<=  const=double(7)  OutDataTypeStr=boolean
  mux : Mux  Inputs=7
  mux1 : Mux  Inputs=7
  rd_{0..4,6} (6 alike) : Delay  DelayLength=double(1)  InitialCondition=0  SampleTime=7.65403750478377e-09
  rd_5 : Delay  DelayLength=double(4)  InitialCondition=0  SampleTime=7.65403750478377e-09
  rd_7 : Delay  DelayLength=double(6)  InitialCondition=0  SampleTime=7.65403750478377e-09
  tappedDelay : Subsystem
  out0 : Outport  OutDataTypeStr=fixdt(1, 50, 37)  SampleTime=7.65403750478377e-09
  out1 : Outport  Port=2  OutDataTypeStr=fixdt(1, 50, 37)  SampleTime=7.65403750478377e-09
  out2 : Outport  Port=3  OutDataTypeStr=fixdt(1, 50, 37)  SampleTime=7.65403750478377e-09
  out3 : Outport  Port=4  OutDataTypeStr=fixdt(1, 50, 37)  SampleTime=7.65403750478377e-09
  out4 : Outport  Port=5  OutDataTypeStr=fixdt(1, 50, 37)  SampleTime=7.65403750478377e-09
  out5 : Outport  Port=6  OutDataTypeStr=fixdt(1, 50, 37)  SampleTime=7.65403750478377e-09
  out6 : Outport  Port=7  OutDataTypeStr=fixdt(1, 50, 37)  SampleTime=7.65403750478377e-09
  wires:
  demux/5 -> out4/1
  demux/2 -> out1/1
  demux/1 -> out0/1
  tappedDelay/1(out0) -> demux/1
  rd_7/1 -> dot_product1_bypass/2(in1)
  Serializer_Subnetwork1/1(out0) -> dot_product_6/2(in2)
  rd_5/1 -> tappedDelay/Enable
  rd_2/1 -> Serializer_Subnetwork1/2(in1)
  rd_1/1 -> Serializer_Subnetwork1/1(in0)
  Serializer_Subnetwork/1(out0) -> dot_product_6/1(in1)
  mux1/1 -> rd_1/1
  counter/1(out0) -> Serializer_Subnetwork/2(in1), rd_2/1
  enb_counter_ge_2_and_enb_counter_le_7/1 -> rd_5/1
  demux/3 -> out2/1
  in13/1 -> mux1/7
  demux/6 -> out5/1
  in11/1 -> mux1/6
  in7/1 -> mux1/4
  in5/1 -> mux1/3
  in3/1 -> mux1/2
  in1/1 -> mux1/1
  rd_6/1 -> dot_product1_bypass/1(in0)
  rd_0/1 -> counter/Enable
  in12/1 -> mux/7
  in9/1 -> mux1/5
  in10/1 -> mux/6
  in8/1 -> mux/5
  dot_product1_bypass/1(out0) -> out6/1
  in4/1 -> mux/3
  in2/1 -> mux/2
  rd_4/1 -> enb_counter_ge_2_and_enb_counter_le_7/2
  in0/1 -> mux/1
  enb_counter_eq_8/1 -> rd_7/1
  in6/1 -> mux/4
  enb_counter_le_6/1 -> rd_0/1
  rd_3/1 -> enb_counter_ge_2_and_enb_counter_le_7/1
  enb_counter_ge_2/1 -> rd_3/1
  demux/4 -> out3/1
  enb_counter_le_7/1 -> rd_4/1
  enb_counter/1 -> enb_counter_le_7/1, enb_counter_le_6/1, enb_counter_ge_2/1, enb_counter_eq_8/1
  mux/1 -> Serializer_Subnetwork/1(in0)
  dot_product_6/1(out1) -> tappedDelay/1(in0), rd_6/1

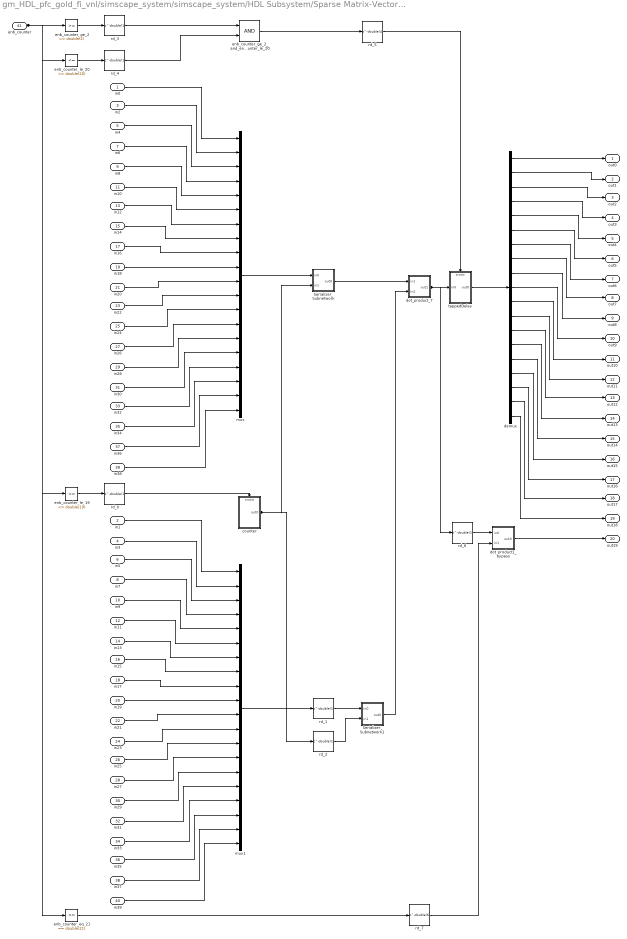
== system gm_HDL_pfc_gold_fi_vnl/simscape_system/simscape_system/HDL Subsystem/Sparse Matrix-Vector Product2/hNNewMatrixC_shared ==
  in0 : Inport  OutDataTypeStr=fixdt(1, 25, 20)  PortDimensions=[7]  SampleTime=7.65403750478377e-09
  in1 : Inport  Port=2  OutDataTypeStr=fixdt(1, 25, 13)  PortDimensions=[7]  SampleTime=7.65403750478377e-09
  in2 : Inport  Port=3  OutDataTypeStr=fixdt(1, 25, 20)  PortDimensions=[7]  SampleTime=7.65403750478377e-09
  in3 : Inport  Port=4  OutDataTypeStr=fixdt(1, 25, 13)  PortDimensions=[7]  SampleTime=7.65403750478377e-09
  in4 : Inport  Port=5  OutDataTypeStr=fixdt(1, 25, 20)  PortDimensions=[7]  SampleTime=7.65403750478377e-09
  in5 : Inport  Port=6  OutDataTypeStr=fixdt(1, 25, 13)  PortDimensions=[7]  SampleTime=7.65403750478377e-09
  in6 : Inport  Port=7  OutDataTypeStr=fixdt(1, 25, 20)  PortDimensions=[7]  SampleTime=7.65403750478377e-09
  in7 : Inport  Port=8  OutDataTypeStr=fixdt(1, 25, 13)  PortDimensions=[7]  SampleTime=7.65403750478377e-09
  in8 : Inport  Port=9  OutDataTypeStr=fixdt(1, 25, 20)  PortDimensions=[7]  SampleTime=7.65403750478377e-09
  in9 : Inport  Port=10  OutDataTypeStr=fixdt(1, 25, 13)  PortDimensions=[7]  SampleTime=7.65403750478377e-09
  in10 : Inport  Port=11  OutDataTypeStr=fixdt(1, 25, 20)  PortDimensions=[7]  SampleTime=7.65403750478377e-09
  in11 : Inport  Port=12  OutDataTypeStr=fixdt(1, 25, 13)  PortDimensions=[7]  SampleTime=7.65403750478377e-09
  in12 : Inport  Port=13  OutDataTypeStr=fixdt(1, 25, 20)  PortDimensions=[7]  SampleTime=7.65403750478377e-09
  in13 : Inport  Port=14  OutDataTypeStr=fixdt(1, 25, 13)  PortDimensions=[7]  SampleTime=7.65403750478377e-09
  in14 : Inport  Port=15  OutDataTypeStr=fixdt(1, 25, 20)  PortDimensions=[7]  SampleTime=7.65403750478377e-09
  in15 : Inport  Port=16  OutDataTypeStr=fixdt(1, 25, 13)  PortDimensions=[7]  SampleTime=7.65403750478377e-09
  in16 : Inport  Port=17  OutDataTypeStr=fixdt(1, 25, 20)  PortDimensions=[7]  SampleTime=7.65403750478377e-09
  in17 : Inport  Port=18  OutDataTypeStr=fixdt(1, 25, 13)  PortDimensions=[7]  SampleTime=7.65403750478377e-09
  in18 : Inport  Port=19  OutDataTypeStr=fixdt(1, 25, 20)  PortDimensions=[7]  SampleTime=7.65403750478377e-09
  in19 : Inport  Port=20  OutDataTypeStr=fixdt(1, 25, 13)  PortDimensions=[7]  SampleTime=7.65403750478377e-09
  in20 : Inport  Port=21  OutDataTypeStr=fixdt(1, 25, 20)  PortDimensions=[7]  SampleTime=7.65403750478377e-09
  in21 : Inport  Port=22  OutDataTypeStr=fixdt(1, 25, 13)  PortDimensions=[7]  SampleTime=7.65403750478377e-09
  in22 : Inport  Port=23  OutDataTypeStr=fixdt(1, 25, 20)  PortDimensions=[7]  SampleTime=7.65403750478377e-09
  in23 : Inport  Port=24  OutDataTypeStr=fixdt(1, 25, 13)  PortDimensions=[7]  SampleTime=7.65403750478377e-09
  in24 : Inport  Port=25  OutDataTypeStr=fixdt(1, 25, 20)  PortDimensions=[7]  SampleTime=7.65403750478377e-09
  in25 : Inport  Port=26  OutDataTypeStr=fixdt(1, 25, 13)  PortDimensions=[7]  SampleTime=7.65403750478377e-09
  in26 : Inport  Port=27  OutDataTypeStr=fixdt(1, 25, 20)  PortDimensions=[7]  SampleTime=7.65403750478377e-09
  in27 : Inport  Port=28  OutDataTypeStr=fixdt(1, 25, 13)  PortDimensions=[7]  SampleTime=7.65403750478377e-09
  in28 : Inport  Port=29  OutDataTypeStr=fixdt(1, 25, 20)  PortDimensions=[7]  SampleTime=7.65403750478377e-09
  in29 : Inport  Port=30  OutDataTypeStr=fixdt(1, 25, 13)  PortDimensions=[7]  SampleTime=7.65403750478377e-09
  in30 : Inport  Port=31  OutDataTypeStr=fixdt(1, 25, 20)  PortDimensions=[7]  SampleTime=7.65403750478377e-09
  in31 : Inport  Port=32  OutDataTypeStr=fixdt(1, 25, 13)  PortDimensions=[7]  SampleTime=7.65403750478377e-09
  in32 : Inport  Port=33  OutDataTypeStr=fixdt(1, 25, 20)  PortDimensions=[7]  SampleTime=7.65403750478377e-09
  in33 : Inport  Port=34  OutDataTypeStr=fixdt(1, 25, 13)  PortDimensions=[7]  SampleTime=7.65403750478377e-09
  in34 : Inport  Port=35  OutDataTypeStr=fixdt(1, 25, 20)  PortDimensions=[7]  SampleTime=7.65403750478377e-09
  in35 : Inport  Port=36  OutDataTypeStr=fixdt(1, 25, 13)  PortDimensions=[7]  SampleTime=7.65403750478377e-09
  in36 : Inport  Port=37  OutDataTypeStr=fixdt(1, 25, 20)  PortDimensions=[7]  SampleTime=7.65403750478377e-09
  in37 : Inport  Port=38  OutDataTypeStr=fixdt(1, 25, 13)  PortDimensions=[7]  SampleTime=7.65403750478377e-09
  in38 : Inport  Port=39  OutDataTypeStr=fixdt(1, 25, 20)  PortDimensions=[7]  SampleTime=7.65403750478377e-09
  in39 : Inport  Port=40  OutDataTypeStr=fixdt(1, 25, 13)  PortDimensions=[7]  SampleTime=7.65403750478377e-09
  enb_counter : Inport  Port=41  OutDataTypeStr=fixdt(0, 7, 0)  SampleTime=7.65403750478377e-09
  Serializer_Subnetwork : Subsystem
  Serializer_Subnetwork1 : Subsystem
  counter : Subsystem
  demux : Demux  Outputs=19
  dot_product1_bypass : Subsystem
  dot_product_7 : Subsystem
  enb_counter_eq_21 : simulink/Logic and Bit Operations/Compare To Constant  relop===  const=double(21)  OutDataTypeStr=boolean
  enb_counter_ge_2 : simulink/Logic and Bit Operations/Compare To Constant  relop=>=  const=double(2)  OutDataTypeStr=boolean
  enb_counter_ge_2_and_enb_counter_le_20 : Logic  AllPortsSameDT=off  OutDataTypeStr=boolean  SampleTime=7.65403750478377e-09
  enb_counter_le_19 : simulink/Logic and Bit Operations/Compare To Constant  relop=<=  const=double(19)  OutDataTypeStr=boolean
  enb_counter_le_20 : simulink/Logic and Bit Operations/Compare To Constant  relop=<=  const=double(20)  OutDataTypeStr=boolean
  mux : Mux  Inputs=20
  mux1 : Mux  Inputs=20
  rd_{0..4,6} (6 alike) : Delay  DelayLength=double(1)  InitialCondition=0  SampleTime=7.65403750478377e-09
  rd_5 : Delay  DelayLength=double(4)  InitialCondition=0  SampleTime=7.65403750478377e-09
  rd_7 : Delay  DelayLength=double(6)  InitialCondition=0  SampleTime=7.65403750478377e-09
  tappedDelay : Subsystem
  out0 : Outport  OutDataTypeStr=fixdt(1, 50, 33)  SampleTime=7.65403750478377e-09
  out1 : Outport  Port=2  OutDataTypeStr=fixdt(1, 50, 33)  SampleTime=7.65403750478377e-09
  out2 : Outport  Port=3  OutDataTypeStr=fixdt(1, 50, 33)  SampleTime=7.65403750478377e-09
  out3 : Outport  Port=4  OutDataTypeStr=fixdt(1, 50, 33)  SampleTime=7.65403750478377e-09
  out4 : Outport  Port=5  OutDataTypeStr=fixdt(1, 50, 33)  SampleTime=7.65403750478377e-09
  out5 : Outport  Port=6  OutDataTypeStr=fixdt(1, 50, 33)  SampleTime=7.65403750478377e-09
  out6 : Outport  Port=7  OutDataTypeStr=fixdt(1, 50, 33)  SampleTime=7.65403750478377e-09
  out7 : Outport  Port=8  OutDataTypeStr=fixdt(1, 50, 33)  SampleTime=7.65403750478377e-09
  out8 : Outport  Port=9  OutDataTypeStr=fixdt(1, 50, 33)  SampleTime=7.65403750478377e-09
  out9 : Outport  Port=10  OutDataTypeStr=fixdt(1, 50, 33)  SampleTime=7.65403750478377e-09
  out10 : Outport  Port=11  OutDataTypeStr=fixdt(1, 50, 33)  SampleTime=7.65403750478377e-09
  out11 : Outport  Port=12  OutDataTypeStr=fixdt(1, 50, 33)  SampleTime=7.65403750478377e-09
  out12 : Outport  Port=13  OutDataTypeStr=fixdt(1, 50, 33)  SampleTime=7.65403750478377e-09
  out13 : Outport  Port=14  OutDataTypeStr=fixdt(1, 50, 33)  SampleTime=7.65403750478377e-09
  out14 : Outport  Port=15  OutDataTypeStr=fixdt(1, 50, 33)  SampleTime=7.65403750478377e-09
  out15 : Outport  Port=16  OutDataTypeStr=fixdt(1, 50, 33)  SampleTime=7.65403750478377e-09
  out16 : Outport  Port=17  OutDataTypeStr=fixdt(1, 50, 33)  SampleTime=7.65403750478377e-09
  out17 : Outport  Port=18  OutDataTypeStr=fixdt(1, 50, 33)  SampleTime=7.65403750478377e-09
  out18 : Outport  Port=19  OutDataTypeStr=fixdt(1, 50, 33)  SampleTime=7.65403750478377e-09
  out19 : Outport  Port=20  OutDataTypeStr=fixdt(1, 50, 33)  SampleTime=7.65403750478377e-09
  wires:
  dot_product1_bypass/1(out0) -> out19/1
  demux/19 -> out18/1
  demux/18 -> out17/1
  demux/17 -> out16/1
  demux/16 -> out15/1
  demux/15 -> out14/1
  demux/14 -> out13/1
  demux/13 -> out12/1
  demux/12 -> out11/1
  demux/11 -> out10/1
  demux/10 -> out9/1
  demux/7 -> out6/1
  demux/6 -> out5/1
  demux/5 -> out4/1
  demux/4 -> out3/1
  rd_6/1 -> dot_product1_bypass/1(in0)
  Serializer_Subnetwork1/1(out0) -> dot_product_7/2(in2)
  Serializer_Subnetwork/1(out0) -> dot_product_7/1(in1)
  demux/3 -> out2/1
  mux1/1 -> rd_1/1
  enb_counter_ge_2_and_enb_counter_le_20/1 -> rd_5/1
  in39/1 -> mux1/20
  in35/1 -> mux1/18
  in31/1 -> mux1/16
  in29/1 -> mux1/15
  in21/1 -> mux1/11
  in19/1 -> mux1/10
  in15/1 -> mux1/8
  dot_product_7/1(out1) -> tappedDelay/1(in0), rd_6/1
  in11/1 -> mux1/6
  demux/1 -> out0/1
  in9/1 -> mux1/5
  in7/1 -> mux1/4
  in1/1 -> mux1/1
  rd_0/1 -> counter/Enable
  in5/1 -> mux1/3
  in27/1 -> mux1/14
  rd_7/1 -> dot_product1_bypass/2(in1)
  in38/1 -> mux/20
  tappedDelay/1(out0) -> demux/1
  in36/1 -> mux/19
  in34/1 -> mux/18
  in3/1 -> mux1/2
  in32/1 -> mux/17
  rd_1/1 -> Serializer_Subnetwork1/1(in0)
  in30/1 -> mux/16
  demux/2 -> out1/1
  in26/1 -> mux/14
  in22/1 -> mux/12
  in20/1 -> mux/11
  in25/1 -> mux1/13
  counter/1(out0) -> rd_2/1, Serializer_Subnetwork/2(in1)
  in18/1 -> mux/10
  rd_2/1 -> Serializer_Subnetwork1/2(in1)
  in16/1 -> mux/9
  in24/1 -> mux/13
  rd_5/1 -> tappedDelay/Enable
  demux/8 -> out7/1
  in14/1 -> mux/8
  in12/1 -> mux/7
  in23/1 -> mux1/12
  in33/1 -> mux1/17
  in8/1 -> mux/5
  in6/1 -> mux/4
  in4/1 -> mux/3
  in2/1 -> mux/2
  in0/1 -> mux/1
  in37/1 -> mux1/19
  rd_3/1 -> enb_counter_ge_2_and_enb_counter_le_20/1
  enb_counter_le_19/1 -> rd_0/1
  mux/1 -> Serializer_Subnetwork/1(in0)
  enb_counter_le_20/1 -> rd_4/1
  enb_counter_ge_2/1 -> rd_3/1
  in10/1 -> mux/6
  rd_4/1 -> enb_counter_ge_2_and_enb_counter_le_20/2
  in28/1 -> mux/15
  in17/1 -> mux1/9
  enb_counter/1 -> enb_counter_le_19/1, enb_counter_ge_2/1, enb_counter_le_20/1, enb_counter_eq_21/1
  in13/1 -> mux1/7
  enb_counter_eq_21/1 -> rd_7/1
  demux/9 -> out8/1
